simulink model "test_learning"  (R2021a)
settings: Solver=FixedStepAuto  StartTime=0.0  StopTime=inf  RelTol=1e-3
undefined symbols (not defined in the file): param1
libraries: simlib_vpc_gp x2
settings Model: Creator=marco  LastModifiedBy=marco

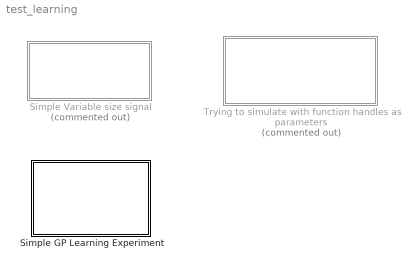
== system test_learning ==
  Simple GP Learning Experiment : Subsystem
  Simple Variable size signal : Subsystem  Commented=on
  Trying to simulate with function handles as parameters : Subsystem  Commented=on

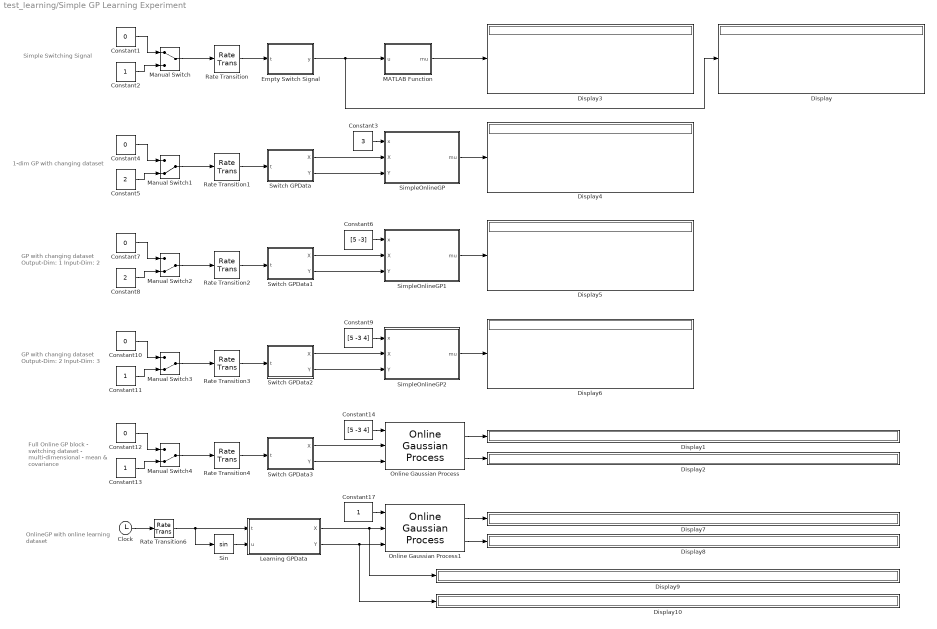
== system test_learning/Simple GP Learning Experiment ==
  note: Simple Switching Signal
  note: 1-dim GP with changing dataset
  note: GP with changing dataset
      | Output-Dim: 1
      | Input-Dim: 2
  note: GP with changing dataset
      | Output-Dim: 2
      | Input-Dim: 3
  note: Full Online GP block
      | - switching dataset
      | - multi-dimensional
      | - mean & covariance
  note: OnlineGP with
      | online learning dataset
  Clock : Clock
  Constant{1,4,7,10,12} (5 alike) : Constant  Value=0
  Constant{2,11,13,17} (4 alike) : Constant
  Constant14 : Constant  Value=[5 -3 4]
  Constant3 : Constant  Value=3
  Constant5 : Constant  Value=2
  Constant6 : Constant  Value=[5 -3]
  Constant8 : Constant  Value=2
  Constant9 : Constant  Value=[5 -3 4]
  Display{,1..10} (11 alike) : Display
  Empty Switch Signal : MATLAB Function  TreatAsAtomicUnit=on
  Learning GPData : MATLAB Function  TreatAsAtomicUnit=on
  MATLAB Function : MATLAB Function  TreatAsAtomicUnit=on
  Manual Switch : ManualSwitch
  Manual Switch{1..4} (4 alike) : ManualSwitch  CurrentSetting=0
  Online Gaussian Process : simlib_vpc_gp/Online Gaussian Process  sn=[0.01 0.01]  kernel=Squared Exponential ARD  hyp=ones(2,4)
      settings: SourceProductName=VPC Library
  Online Gaussian Process1 : simlib_vpc_gp/Online Gaussian Process  sn=0.01  kernel=Squared Exponential ARD  hyp=[1 1]
      settings: SourceProductName=VPC Library
  Rate Transition{,1..4,6} (6 alike) : RateTransition  OutPortSampleTime=0.1
  SimpleOnlineGP : MATLAB Function  TreatAsAtomicUnit=on
  SimpleOnlineGP1 : MATLAB Function  TreatAsAtomicUnit=on
  SimpleOnlineGP2 : MATLAB Function  TreatAsAtomicUnit=on
  Sin : Trigonometry
  Switch GPData : MATLAB Function  TreatAsAtomicUnit=on
  Switch GPData1 : MATLAB Function  TreatAsAtomicUnit=on
  Switch GPData2 : MATLAB Function  TreatAsAtomicUnit=on
  Switch GPData3 : MATLAB Function  TreatAsAtomicUnit=on
  wires:
  Online Gaussian Process/1 -> Display1/1
  Online Gaussian Process/2 -> Display2/1
  MATLAB Function/1(mu) -> Display3/1
  Manual Switch/1 -> Rate Transition/1
  Empty Switch Signal/1(y) -> Display/1, MATLAB Function/1(u)
  Rate Transition/1 -> Empty Switch Signal/1(t)
  Constant2/1 -> Manual Switch/2
  Constant1/1 -> Manual Switch/1
  SimpleOnlineGP/1(mu) -> Display4/1
  Constant3/1 -> SimpleOnlineGP/1(x)
  Manual Switch1/1 -> Rate Transition1/1
  Rate Transition1/1 -> Switch GPData/1(t)
  Constant5/1 -> Manual Switch1/2
  Constant4/1 -> Manual Switch1/1
  Switch GPData/1(X) -> SimpleOnlineGP/2(X)
  Switch GPData/2(Y) -> SimpleOnlineGP/3(Y)
  SimpleOnlineGP1/1(mu) -> Display5/1
  Constant6/1 -> SimpleOnlineGP1/1(x)
  Manual Switch2/1 -> Rate Transition2/1
  Constant8/1 -> Manual Switch2/2
  Rate Transition2/1 -> Switch GPData1/1(t)
  Constant7/1 -> Manual Switch2/1
  Switch GPData1/1(X) -> SimpleOnlineGP1/2(X)
  Switch GPData1/2(Y) -> SimpleOnlineGP1/3(Y)
  Rate Transition3/1 -> Switch GPData2/1(t)
  Manual Switch3/1 -> Rate Transition3/1
  Switch GPData2/2(Y) -> SimpleOnlineGP2/3(Y)
  Switch GPData2/1(X) -> SimpleOnlineGP2/2(X)
  SimpleOnlineGP2/1(mu) -> Display6/1
  Constant10/1 -> Manual Switch3/1
  Constant11/1 -> Manual Switch3/2
  Constant9/1 -> SimpleOnlineGP2/1(x)
  Rate Transition4/1 -> Switch GPData3/1(t)
  Switch GPData3/1(X) -> Online Gaussian Process/2
  Switch GPData3/2(Y) -> Online Gaussian Process/3
  Manual Switch4/1 -> Rate Transition4/1
  Constant12/1 -> Manual Switch4/1
  Constant14/1 -> Online Gaussian Process/1
  Constant13/1 -> Manual Switch4/2
  Clock/1 -> Rate Transition6/1
  Online Gaussian Process1/1 -> Display7/1
  Online Gaussian Process1/2 -> Display8/1
  Learning GPData/1(X) -> Display9/1, Online Gaussian Process1/2
  Constant17/1 -> Online Gaussian Process1/1
  Learning GPData/2(Y) -> Display10/1, Online Gaussian Process1/3
  Sin/1 -> Learning GPData/2(u)
  Rate Transition6/1 -> Learning GPData/1(t), Sin/1

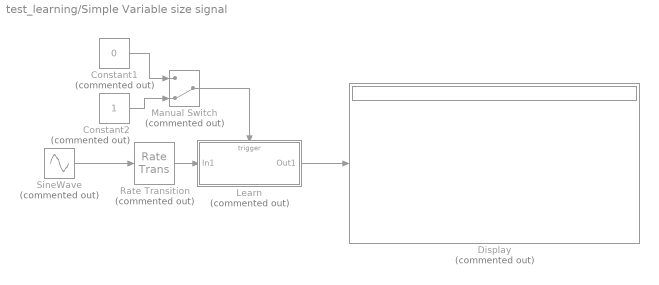
== system test_learning/Simple Variable size signal ==
  Constant1 : Constant  Commented=on  Value=0
  Constant2 : Constant  Commented=on
  Display : Display  Commented=on
  Learn : Subsystem  Commented=on  TreatAsAtomicUnit=on
  Manual Switch : ManualSwitch  Commented=on  CurrentSetting=0
  Rate Transition : RateTransition  Commented=on  OutPortSampleTime=0.1
  SineWave : Sin  Commented=on  SampleTime=0
  wires:
  Rate Transition/1 -> Learn/1(In1)
  Manual Switch/1 -> Learn/Trigger
  Constant2/1 -> Manual Switch/2
  Learn/1(Out1) -> Display/1
  Constant1/1 -> Manual Switch/1
  SineWave/1 -> Rate Transition/1

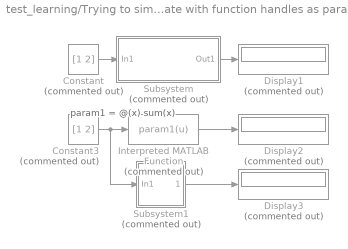
== system test_learning/Trying to simulate with function handles as parameters ==
  note: param1 = @(x) sum(x)
  Constant : Constant  Commented=on  Value=[1 2]
  Constant3 : Constant  Commented=on  Value=[1 2]
  Display1 : Display  Commented=on
  Display2 : Display  Commented=on
  Display3 : Display  Commented=on
  Interpreted MATLAB Function : MATLABFcn  Commented=on  MATLABFcn=param1(u)
  Subsystem : Subsystem  Commented=on  mask{param1="@(x) sum(x)"}
  Subsystem1 : Subsystem  Commented=on  TreatAsAtomicUnit=on  mask{param1=feval(param1,u)}
      mask prompts: param1 "Simulink:blkprm_prompts:MATLABFcnFunction"
      mask TypeOptions param1:
      | Interpreted MATLAB
      | Function/MATLABFcn
      mask DialogControl param1 Prompt: MATLAB function:
  wires:
  Constant3/1 -> Subsystem1/1(In1), Interpreted MATLAB Function/1
  Interpreted MATLAB Function/1 -> Display2/1
  Subsystem/1(Out1) -> Display1/1
  Subsystem1/1(Out1) -> Display3/1
  Constant/1 -> Subsystem/1(In1)

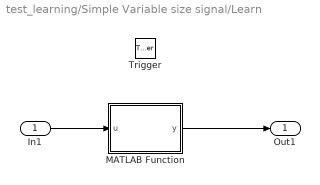
== system test_learning/Simple Variable size signal/Learn ==
  In1 : Inport
  Trigger : TriggerPort  VariantControl=(inherit)
  MATLAB Function : MATLAB Function  TreatAsAtomicUnit=on
  Out1 : Outport
  wires:
  In1/1 -> MATLAB Function/1(u)
  MATLAB Function/1(y) -> Out1/1

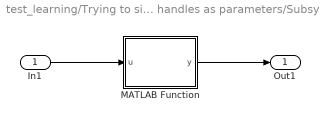
== system test_learning/Trying to simulate with function handles as parameters/Subsystem ==
  In1 : Inport
  MATLAB Function : MATLAB Function  TreatAsAtomicUnit=on
  Out1 : Outport
  wires:
  In1/1 -> MATLAB Function/1(u)
  MATLAB Function/1(y) -> Out1/1

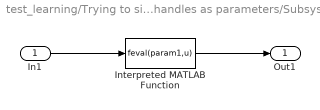
== system test_learning/Trying to simulate with function handles as parameters/Subsystem1 ==
  In1 : Inport
  Interpreted MATLAB Function : MATLABFcn  MATLABFcn=feval(param1,u)
  Out1 : Outport
  wires:
  In1/1 -> Interpreted MATLAB Function/1
  Interpreted MATLAB Function/1 -> Out1/1

== matlab function test_learning/Trying to simulate with function handles as parameters/Subsystem/MATLAB Function ==
  data: u input; y output; param1 parameter string
function y = fcn(u, param1)
disp(param1)
y = u;

== matlab function test_learning/Simple Variable size signal/Learn/MATLAB Function ==
  data: u input; y output size=[1 10]
function y = fcn(u)

persistent data
if isempty(data)
    data = [];
end

coder.varsize('y',[1 10]);

% learn new data point
data = [data u];

y = data;

== matlab function test_learning/Simple GP Learning Experiment/Learning GPData ==
  data: X output size=[10 1]; t input; Y output size=[10 1]; u input
function [X,Y] = onlinelearndata(t,u) %#codegen
T = 5; % Time when a datapoint is added
M = 10; % how many datapoints

% define persistent data
persistent X_ Y_
coder.varsize('X_',[M 1])
coder.varsize('Y_',[M 1])

% init data
if isempty(X_) || isempty(Y_)
    X_ = zeros(0,1);
    Y_ = zeros(0,1);
end

% append datapoint if triggered
if mod(t,T) == 0
    if length(X_) < M
        X_ = [X_; u];
        Y_ = [Y_; 2*u];
    else
        X_ = [X_(2:M); u];
        Y_ = [Y_(2:M); 2*u];
    end
end

% set output
X = X_;
Y = Y_;

end

== matlab function test_learning/Simple GP Learning Experiment/MATLAB Function ==
  data: u input; mu output size=[1 10]
function mu = fcn(u) %#codegen
% persistent U A
% 
% coder.varsize('A',[10 6]);
% 
% if isempty(U)
%     U = u;
%     %A = [];
%     A = zeros(0,6);
% end
% 
% y = U;

persistent A U

if isempty(U)
    U = u;
end

coder.varsize('A');
% if isempty(A)
%     
% end

% update internal copies of U data if they have changed
if ~isequal(U,u)
    U = u;
    
    % clear A
    A = zeros(0,1);
end

% Calculate output
mu = 0;
if ~isempty(U)
    % init A matrix
    if isempty(A)
        M = length(u);
        A = zeros(M,1);
    end
end

end

== matlab function test_learning/Simple GP Learning Experiment/Empty Switch Signal ==
  data: y output size=[1 10]; t input
function y = fcn(t)
y = [];
if t >= 1
    y = 1;
end
end

== matlab function test_learning/Simple GP Learning Experiment/SimpleOnlineGP ==
  data: x input; mu output; X input; Y input
function mu = simple_online_gp(x, X, Y) %#codegen
% persistent U A
% 
% coder.varsize('A',[10 6]);
% 
% if isempty(U)
%     U = u;
%     %A = [];
%     A = zeros(0,6);
% end
% 
% y = U;

persistent Kinv A X_ Y_

% init internal copy of I/O Data if not yet initialized
if isempty(X_) || isempty(Y_)
    X_ = X; Y_ = Y;
end

coder.varsize('Kinv');
coder.varsize('A');
% if isempty(A)
%     
% end

% update internal copies of data if they have changed
if ~isequal(X_,X) || ~isequal(Y_,Y)
    X_ = X; Y_ = Y;
    
    % clear Kinv and A
    A = zeros(0,1);
    Kinv = zeros(0,0);
end

% Calculate output
mu = 0;
if ~isempty(X_) && ~isempty(Y_)
    % define kernel-function
    kernelfun = @SEARD;
    
    % init inverse K and A matrices if not yet initialized
    if isempty(Kinv) || isempty(A)
        M = length(X_);
        A = zeros(M,1);
        Kinv = zeros(M,M);
        
        Kinv(:,:) = inv(kernelfun(X,X,[1 1]) + 0.01^2*eye(M));
        A(:) = Kinv(:,:) * Y(:);
    end
    
    % calculate GP output
    [mu, ~] = gp_calc(x, X, Y, kernelfun, 0.01, [1 1], Kinv, A);
%     mu(1:end) = mu_(1:end);
end

end

== matlab function test_learning/Simple GP Learning Experiment/Switch GPData ==
  data: X output size=[10 1]; t input; Y output size=[10 1]
function [X,Y] = fcn(t)
X = zeros(0,1);
Y = zeros(0,1);
if t == 1
    X = 1;
    Y = 2;
end
if t == 2
    X = [1; 3; 5];
    Y = [2; 6; 10];
end

end

== matlab function test_learning/Simple GP Learning Experiment/SimpleOnlineGP1 ==
  data: x input; mu output; X input; Y input
function mu = simple_online_gp(x, X, Y) %#codegen

persistent Kinv A X_ Y_

% init internal copy of I/O Data if not yet initialized
if isempty(X_) || isempty(Y_)
    X_ = X; Y_ = Y;
end

coder.varsize('Kinv');
coder.varsize('A');
% if isempty(A)
%     
% end

% update internal copies of data if they have changed
if ~isequal(X_,X) || ~isequal(Y_,Y)
    X_ = X; Y_ = Y;
    
    % clear Kinv and A
    A = zeros(0,1);
    Kinv = zeros(0,0);
end

% Calculate output
mu = 0;
if ~isempty(X_) && ~isempty(Y_)
    % define kernel-function
    kernelfun = @SEARD;
    
%     N = length(x);
    [M, N] = size(X_);
    
    % init inverse K and A matrices if not yet initialized
    if isempty(Kinv) || isempty(A)
%         [M, ~] = size(X_);
        A = zeros(M,1);
        Kinv = zeros(M,M);
        
        Kinv(:,:) = inv(kernelfun(X,X,ones(1,N+1)) + 0.01^2*eye(M));
        A(:) = Kinv(:,:) * Y(:);
    end
    
    % calculate GP output
    [mu, ~] = gp_calc(x, X, Y, kernelfun, 0.01, ones(1,N+1), Kinv, A);
%     mu(1:end) = mu_(1:end);
end

end

== matlab function test_learning/Simple GP Learning Experiment/Switch GPData1 ==
  data: X output size=[10 2]; t input; Y output size=[10 1]
function [X,Y] = fcn(t)
X = zeros(0,2);
Y = zeros(0,1);

%coder.varsize('X',[10,2],[1,0]);
if t == 1
    X = [1 2];
    Y = 2;
end
if t == 2
    X = [1 2; 3 0; 5 -3];
    Y = [2; 6; 10];
end

end

== matlab function test_learning/Simple GP Learning Experiment/SimpleOnlineGP2 ==
  data: x input; mu output; X input; Y input
function mu = simple_online_gp(x, X, Y) %#codegen

persistent Kinv A X_ Y_

% init internal copy of I/O Data if not yet initialized
if isempty(X_) || isempty(Y_)
    X_ = X; Y_ = Y;
end

coder.varsize('Kinv');
coder.varsize('A');

% Q = size(Y,2); % this doesn't work, but we know the dimension from sn anyway -> so no problem!
Q = 2;

% update internal copies of data if they have changed
if ~isequal(X_,X) || ~isequal(Y_,Y)
    X_ = X; Y_ = Y;
    
    % clear Kinv and A
    A = zeros(0,Q);
    Kinv = zeros(0,0,Q);
end

% Calculate output
mu = zeros(Q,1);
if ~isempty(X_) && ~isempty(Y_)
    % define kernel-function
    kernelfun = @SEARD;
    
    % init inverse K and A matrices if not yet initialized
    [M, N] = size(X_);
    if isempty(Kinv) || isempty(A)
        A = zeros(M,Q);
        Kinv = zeros(M,M,Q);
        
        for i=1:Q
            Kinv(:,:,i) = inv(kernelfun(X,X,ones(1,N+1)) + 0.01^2*eye(M));
            A(:,i) = Kinv(:,:,i) * Y(:,i);
        end
    end
    
    % calculate GP output
    [mu, ~] = gp_calc(x, X, Y, kernelfun, [0.01 0.01], ones(Q,N+1), Kinv, A);
end

end

== matlab function test_learning/Simple GP Learning Experiment/Switch GPData2 ==
  data: X output size=[10 3]; t input; Y output size=[10 2]
function [X,Y] = fcn(t)
X = zeros(0,3);
Y = zeros(0,2);

if t == 1
    X = [1 2 3];
    Y = [2 3];
end
if t == 2
    X = [1 2 3; 3 0 1; 5 -3 4];
    Y = [2 1; 6 0; 10 7];
end

end

== matlab function test_learning/Simple GP Learning Experiment/Switch GPData3 ==
  data: X output size=[10 3]; t input; Y output size=[10 2]
function [X,Y] = fcn(t)
X = zeros(0,3);
Y = zeros(0,2);

if t == 1
    X = [1 2 3];
    Y = [2 3];
end
if t == 2
    X = [1 2 3; 3 0 1; 5 -3 4];
    Y = [2 1; 6 0; 10 7];
end

end
